simulink model "IIC_assignment_1"  (R2017a)
settings: Solver=VariableStepAuto  StartTime=0.0  StopTime=20  RelTol=1e-3
values from neighbouring files (symbols this model uses):
  A = (1/tau)*[-(1+d) 1 0;d -(1+d) 1;0 d -(1+d)]    [IIC_param.m]
  B = (1/tau)*[0 k -k;0 0 0;1 0 0]    [IIC_param.m]
  C = [1 0 0;0 0 a]    [IIC_param.m]
libraries: simulink x2
settings Model: Creator=Dr.Saraf  LastModifiedBy=Dr.Saraf

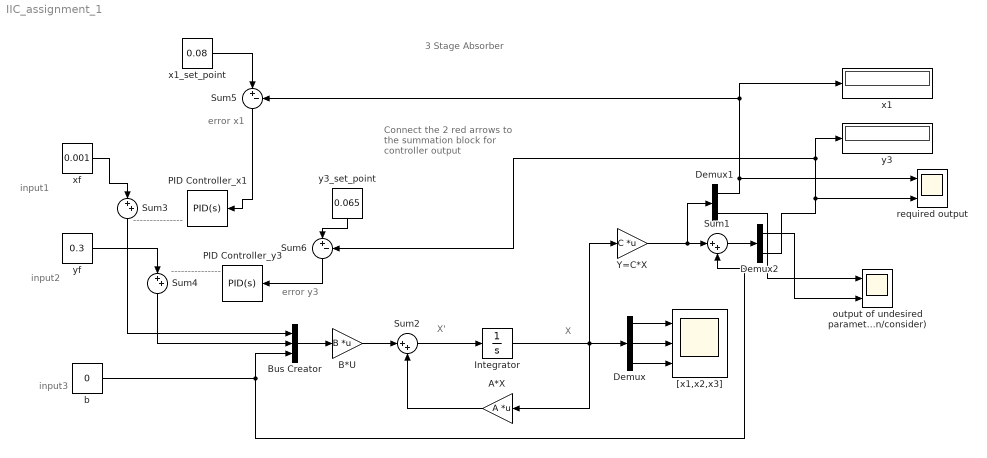
== system IIC_assignment_1 ==
  note: ---------------
  note: Connect the 2 red arrows
      | to the summation block
      | for controller output
  note: 3 Stage Absorber
  note: error x1
  note: error y3
  note: input3
  note: input2
  note: input1
  note: X
  note: X'
  note: ---------------
  A*X : Gain  Gain=A  Multiplication=Matrix(K*u)
  B*U : Gain  Gain=B  Multiplication=Matrix(K*u)
  Bus Creator : BusCreator  Inputs=3
  Demux : Demux  Outputs=3
  Demux1 : Demux  Outputs=2
  Demux2 : Demux  Outputs=2
  Integrator : Integrator
  PID Controller_x1 : simulink/Continuous/PID Controller  Controller=PID  TimeDomain=Continuous-time  SampleTime=-1  IntegratorMethod=Forward Euler  FilterMethod=Forward Euler  Form=Parallel  UseFilter=on  ControllerParametersSource=internal  P=10.5934216097695  I=2.45026379628214  D=11.21528401845  N=71.0520680214784  InitialConditionSource=internal  InitialConditionForIntegrator=0  InitialConditionForFilter=0  ExternalReset=none  LimitOutput=off  UpperSaturationLimit=inf  LowerSaturationLimit=-inf  LinearizeAsGain=on  AntiWindupMode=none  Kb=1  TrackingMode=off  Kt=1  PParamMin=[]  PParamMax=[]  IParamMin=[]  IParamMax=[]  DParamMin=[]  DParamMax=[]  NParamMin=[]  NParamMax=[]  KbParamMin=[]  KbParamMax=[]  KtParamMin=[]  KtParamMax=[]  POutMin=[]  POutMax=[]  IOutMin=[]  IOutMax=[]  DOutMin=[]  DOutMax=[]  NOutMin=[]  NOutMax=[]  KbOutMin=[]  KbOutMax=[]  KtOutMin=[]  KtOutMax=[]  IntegratorOutMin=[]  IntegratorOutMax=[]  FilterOutMin=[]  FilterOutMax=[]  SumOutMin=[]  SumOutMax=[]  SumI1OutMin=[]  SumI1OutMax=[]  SumI2OutMin=[]  SumI2OutMax=[]  SumI3OutMin=[]  SumI3OutMax=[]  SumDOutMin=[]  SumDOutMax=[]  SaturationOutMin=[]  SaturationOutMax=[]  IntegratorContinuousStateAttributes=''  IntegratorStateMustResolveToSignalObject=off  IntegratorRTWStateStorageClass=Auto  FilterContinuousStateAttributes=''  FilterStateMustResolveToSignalObject=off  FilterRTWStateStorageClass=Auto  DifferentiatorICPrevScaledInput=0  DifferentiatorOutMin=[]  DifferentiatorOutMax=[]  InitialConditionSetting=State (most efficient)
  PID Controller_y3 : simulink/Continuous/PID Controller  Controller=PID  TimeDomain=Continuous-time  SampleTime=-1  IntegratorMethod=Forward Euler  FilterMethod=Forward Euler  Form=Parallel  UseFilter=on  ControllerParametersSource=internal  P=-1.84577405431843  I=-4.76589515643767  D=0.00295864753653049  N=623.857364396609  InitialConditionSource=internal  InitialConditionForIntegrator=0  InitialConditionForFilter=0  ExternalReset=none  LimitOutput=off  UpperSaturationLimit=inf  LowerSaturationLimit=-inf  LinearizeAsGain=on  AntiWindupMode=none  Kb=1  TrackingMode=off  Kt=1  PParamMin=[]  PParamMax=[]  IParamMin=[]  IParamMax=[]  DParamMin=[]  DParamMax=[]  NParamMin=[]  NParamMax=[]  KbParamMin=[]  KbParamMax=[]  KtParamMin=[]  KtParamMax=[]  POutMin=[]  POutMax=[]  IOutMin=[]  IOutMax=[]  DOutMin=[]  DOutMax=[]  NOutMin=[]  NOutMax=[]  KbOutMin=[]  KbOutMax=[]  KtOutMin=[]  KtOutMax=[]  IntegratorOutMin=[]  IntegratorOutMax=[]  FilterOutMin=[]  FilterOutMax=[]  SumOutMin=[]  SumOutMax=[]  SumI1OutMin=[]  SumI1OutMax=[]  SumI2OutMin=[]  SumI2OutMax=[]  SumI3OutMin=[]  SumI3OutMax=[]  SumDOutMin=[]  SumDOutMax=[]  SaturationOutMin=[]  SaturationOutMax=[]  IntegratorContinuousStateAttributes=''  IntegratorStateMustResolveToSignalObject=off  IntegratorRTWStateStorageClass=Auto  FilterContinuousStateAttributes=''  FilterStateMustResolveToSignalObject=off  FilterRTWStateStorageClass=Auto  DifferentiatorICPrevScaledInput=0  DifferentiatorOutMin=[]  DifferentiatorOutMax=[]  InitialConditionSetting=State (most efficient)
  Sum{1..4} (4 alike) : Sum  Inputs=|++
  Sum5 : Sum  Inputs=|+-
  Sum6 : Sum  Inputs=|+-
  Y=C*X : Gain  Gain=C  Multiplication=Matrix(K*u)
  "[x1,x2,x3]" : Scope  NumInputPorts=3
  b : Constant  Value=0
  output of undesired parameters (Dont open/consider) : Scope  NumInputPorts=2
  "required output " : Scope  NumInputPorts=2
  x1 : Display
  "x1_set_point " : Constant  Value=0.08
  xf : Constant  Value=0.001
  y3 : Display
  y3_set_point : Constant  Value=0.065
  yf : Constant  Value=0.3
  wires:
  Demux/2 -> "[x1,x2,x3]"/2
  Bus Creator/1 -> B*U/1
  Demux2/1 -> output of undesired parameters (Dont open/consider)/2
  B*U/1 -> Sum2/1
  Demux/1 -> "[x1,x2,x3]"/1
  Sum1/1 -> Demux2/1
  Demux/3 -> "[x1,x2,x3]"/3
  b/1 -> Bus Creator/3, Sum1/2
  Y=C*X/1 -> Demux1/1, Sum1/1
  Sum2/1 -> Integrator/1
  Integrator/1 -> Y=C*X/1, Demux/1, A*X/1
  A*X/1 -> Sum2/2
  Demux1/2 -> output of undesired parameters (Dont open/consider)/1
  Demux1/1 -> "required output "/1, x1/1, Sum5/2
  yf/1 -> Sum4/1
  xf/1 -> Sum3/1
  Sum3/1 -> Bus Creator/1
  Sum4/1 -> Bus Creator/2
  Demux2/2 -> Sum6/2, y3/1, "required output "/2
  "x1_set_point "/1 -> Sum5/1
  Sum5/1 -> PID Controller_x1/1
  Sum6/1 -> PID Controller_y3/1
  y3_set_point/1 -> Sum6/1
